simulink model "Diff_rovnice"  (R2014a)
settings: Solver=ode45  StartTime=0.0  StopTime=10.0  RelTol=1e-3
values from neighbouring files (symbols this model uses):
  B = 0.01    [AAACviko_05.m]    (also in crit_fun2.m; uloha1.m)
  g = 9.81    [AAACviko_05.m]    (also in crit_fun2.m; uloha1.m)
  J = m*l^2    (= 0.032)    [AAACviko_05.m]    (also in crit_fun2.m; uloha1.m)
  l = 0.4    [AAACviko_05.m]    (also in crit_fun2.m; uloha1.m)
  m = 0.2    [AAACviko_05.m]    (also in crit_fun2.m; gennumbers.m = 10; uloha1.m)
settings Model: Creator=tomas  LastModifiedBy=tomas

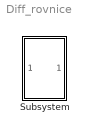
== system Diff_rovnice ==
  Subsystem : Subsystem
  wires:
  ? -> Subsystem/1(In1)

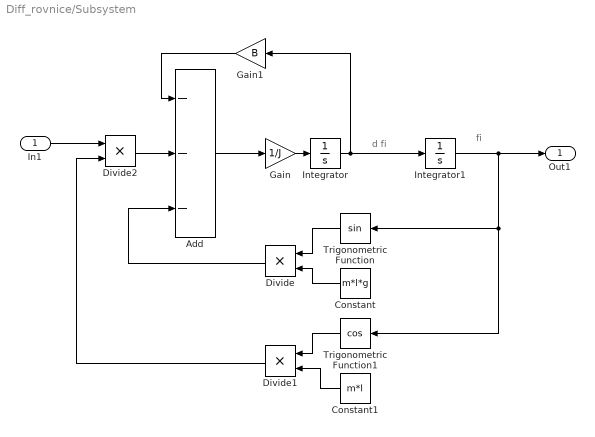
== system Diff_rovnice/Subsystem ==
  note: fi
  note: d fi
  In1 : Inport
  Add : Sum  Inputs=---
  Constant : Constant  Value=m*l*g
  Constant1 : Constant  Value=m*l
  Divide : Product  Inputs=**
  Divide1 : Product  Inputs=**
  Divide2 : Product  Inputs=**
  Gain : Gain  Gain=1/J
  Gain1 : Gain  Gain=B
  Integrator : Integrator
  Integrator1 : Integrator
  Trigonometric Function : Trigonometry
  Trigonometric Function1 : Trigonometry  Operator=cos
  Out1 : Outport
  wires:
  Integrator/1 -> Gain1/1, Integrator1/1
  Add/1 -> Gain/1
  Trigonometric Function1/1 -> Divide1/1
  Constant/1 -> Divide/2
  Gain/1 -> Integrator/1
  Trigonometric Function/1 -> Divide/1
  Constant1/1 -> Divide1/2
  Divide/1 -> Add/3
  Gain1/1 -> Add/1
  Integrator1/1 -> Out1/1, Trigonometric Function1/1, Trigonometric Function/1
  Divide2/1 -> Add/2
  Divide1/1 -> Divide2/2
  In1/1 -> Divide2/1
